simulink model "Q5_W1"  (R2020b)
settings: Solver=VariableStepAuto  StartTime=0.0  StopTime=10  RelTol=1e-3
settings Model: Creator=hp  LastModifiedBy=hp

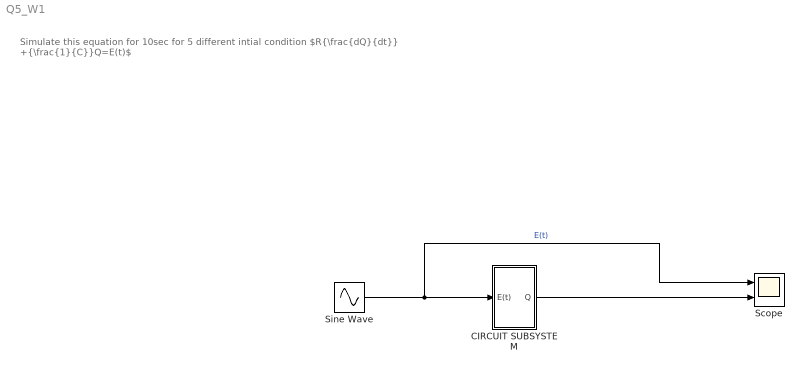
== system Q5_W1 ==
  note: Simulate this equation for 10sec for 5 different intial condition
      | $R{\frac{dQ}{dt}} +{\frac{1}{C}}Q=E(t)$
  CIRCUIT SUBSYSTEM : Subsystem
  Scope : Scope  NumInputPorts=2
  Sine Wave : Sin  SampleTime=0
  wires:
  Sine Wave/1 -> Scope/1, CIRCUIT SUBSYSTEM/1(E(t))  "E(t)"
  CIRCUIT SUBSYSTEM/1(Q) -> Scope/2

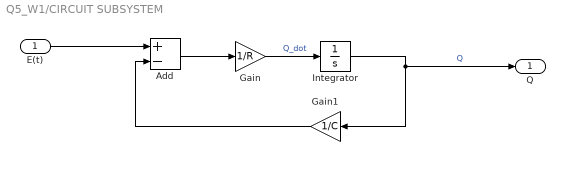
== system Q5_W1/CIRCUIT SUBSYSTEM ==
  E(t) : Inport
  Add : Sum  Inputs=+-
  Gain : Gain  Gain=1/R  mask{R=0.1}
  Gain1 : Gain  Gain=1/C  mask{C=100000}
      mask prompts: C "1/C"
  Integrator : Integrator
  Q : Outport
  wires:
  Integrator/1 -> Q/1, Gain1/1  "Q"
  Gain1/1 -> Add/2
  E(t)/1 -> Add/1
  Add/1 -> Gain/1
  Gain/1 -> Integrator/1  "Q_dot"
